simulink subsystem "Mi_Piero"  (R2024b)
settings: Solver=VariableStepAuto  StartTime=0.0  StopTime=10.0  RelTol=1e-3
settings Model: Creator=Chenfu  LastModifiedBy=Chenfu

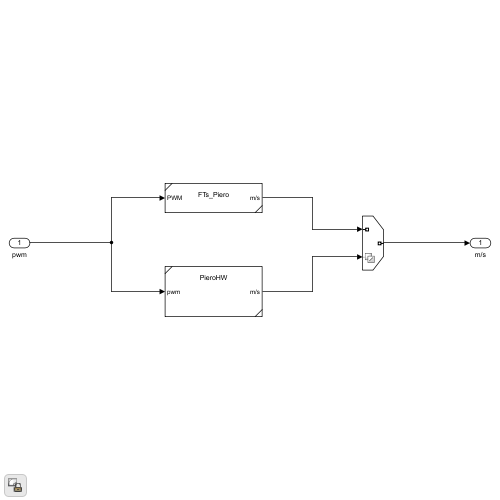
[thumbnail: Simulink's stored preview of the top-level diagram]
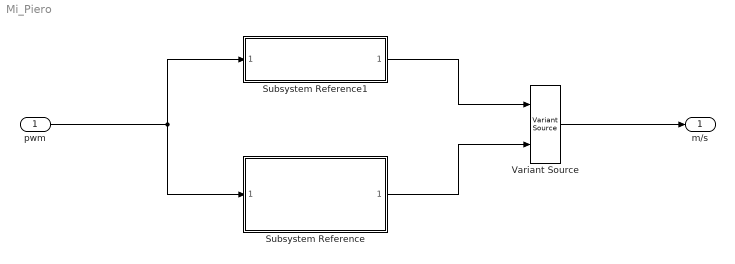
== system Mi_Piero ==
  pwm : Inport
  Subsystem Reference : Subsystem  ReferencedSubsystem=PieroHW
  Subsystem Reference1 : Subsystem  ReferencedSubsystem=FTs_Piero
  Variant Source : VariantSource  VariantControlMode=sim codegen switching
  m/s : Outport
  wires:
  pwm/1 -> Subsystem Reference/1, Subsystem Reference1/1
  Subsystem Reference1/1 -> Variant Source/1
  Subsystem Reference/1 -> Variant Source/2
  Variant Source/1 -> m/s/1
